simulink model "ComparacionControladores"  (R2021a)
settings: Solver=VariableStepAuto  StartTime=0.0  StopTime=480  MaxStep=200.0  RelTol=1e-3
values from neighbouring files (symbols this model uses):
  h0 = 0.45    [practica4.m]
  k = 3.1623    [practica4.m]
  p = 0.00237    [practica4.m]
  Ts = 1    [practica4.m]
  u0 = Qi / (A_sal * sqrt(2 * g * h0))    [practica4.m]
libraries: cstblocks x5
settings Model: Creator=faust  LastModifiedBy=faust

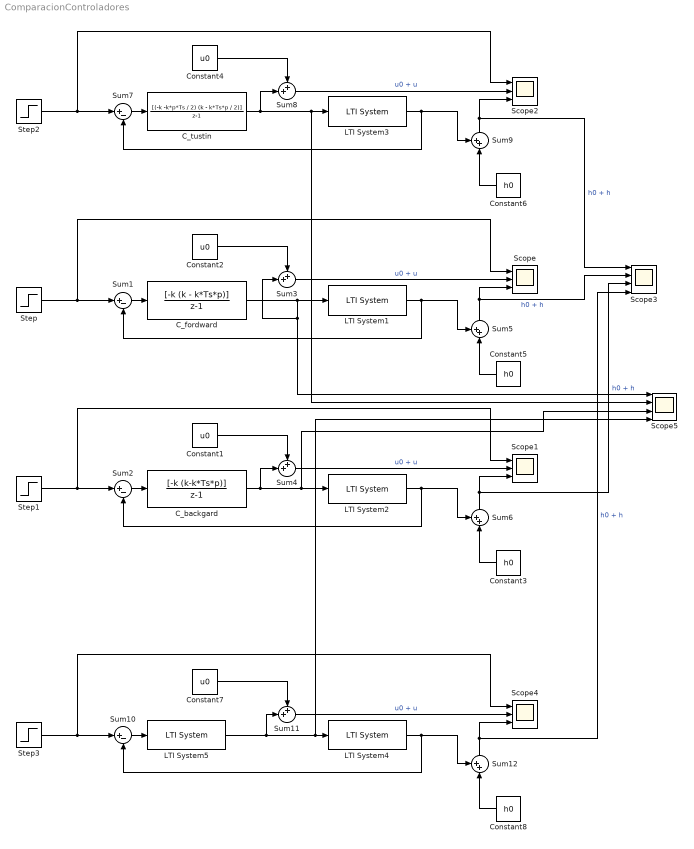
== system ComparacionControladores ==
  C_backgard : DiscreteTransferFcn  Numerator=[-k (k-k*Ts*p)]  Denominator=[1 -1]  SampleTime=1
  C_fordward : DiscreteTransferFcn  Numerator=[-k (k - k*Ts*p)]  Denominator=[1 -1]  SampleTime=1
  C_tustin : DiscreteTransferFcn  Numerator=[(-k -k*p*Ts / 2) (k - k*Ts*p / 2)]  Denominator=[1 -1]  InitialStates=0.5  SampleTime=1
  Constant{1..2,4,7} (4 alike) : Constant  Value=u0
  Constant{3,5..6,8} (4 alike) : Constant  Value=h0
  LTI System{1..4} (4 alike) : cstblocks/LTI System  sys=P  IC=[]
  LTI System5 : cstblocks/LTI System  sys=C  IC=[]
  Scope{,1..2,4} (4 alike) : Scope  NumInputPorts=3
  Scope3 : Scope  NumInputPorts=4
  Scope5 : Scope  NumInputPorts=4
  Step{,1..3} (4 alike) : Step  Time=10  After=0.1  SampleTime=0
  Sum{1..2,7,10} (4 alike) : Sum  Inputs=|+-
  Sum{3..6,8..9,11..12} (8 alike) : Sum  Inputs=++|
  wires:
  Sum3/1 -> Scope/2  "u0 + u"
  Sum5/1 -> Scope3/2, Scope/3  "h0 + h"
  Sum1/1 -> C_fordward/1
  Step/1 -> Scope/1, Sum1/1
  Constant2/1 -> Sum3/1
  LTI System1/1 -> Sum1/2, Sum5/1
  C_fordward/1 -> Scope5/1, Sum3/2, LTI System1/1
  Constant5/1 -> Sum5/2
  C_backgard/1 -> Sum4/2, Scope5/3, LTI System2/1
  Sum2/1 -> C_backgard/1
  Constant3/1 -> Sum6/2
  LTI System2/1 -> Sum2/2, Sum6/1
  Constant1/1 -> Sum4/1
  Sum6/1 -> Scope3/3, Scope1/3  "h0 + h"
  Step1/1 -> Scope1/1, Sum2/1
  Sum4/1 -> Scope1/2  "u0 + u"
  C_tustin/1 -> Sum8/2, Scope5/2, LTI System3/1
  Sum7/1 -> C_tustin/1
  Constant6/1 -> Sum9/2
  LTI System3/1 -> Sum7/2, Sum9/1
  Constant4/1 -> Sum8/1
  Sum9/1 -> Scope2/3, Scope3/1  "h0 + h"
  Step2/1 -> Scope2/1, Sum7/1
  Sum8/1 -> Scope2/2  "u0 + u"
  Constant8/1 -> Sum12/2
  Sum11/1 -> Scope4/2  "u0 + u"
  Sum10/1 -> LTI System5/1
  Step3/1 -> Scope4/1, Sum10/1
  LTI System4/1 -> Sum10/2, Sum12/1
  Sum12/1 -> Scope3/4, Scope4/3  "h0 + h"
  Constant7/1 -> Sum11/1
  LTI System5/1 -> Sum11/2, Scope5/4, LTI System4/1
